simulink model "stage1_ball_joint_pd_uniform"  (R2025b)
settings: Solver=FixedStepDiscrete  StartTime=0.0  StopTime=stop_time_s  FixedStep=dt_sim  RelTol=1e-3
PostLoadFcn:
  | evalin('base', 'run(fullfile(fileparts(get_param(''stage1_ball_joint_pd_uniform'', ''FileName'')), ''init_stage1_ball_joint_pd_workspace.m''))')
InitFcn:
  | evalin('base', 'run(fullfile(fileparts(get_param(''stage1_ball_joint_pd_uniform'', ''FileName'')), ''init_stage1_ball_joint_pd_workspace.m''))')
values from neighbouring files (symbols this model uses):
  alpha_v = 1 - exp(-dt_ctrl / tau_v)    [init_stage1_ball_joint_pd_workspace.m]    (also in simulate_uniform_ball_joint_pd.m = 1 - exp(-dt_ctrl / params.tau_v))
  B_axis = 0.5    [init_stage1_ball_joint_pd_workspace.m]
  dt_ctrl = 1 / 60    (= 0.0166666666667)    [init_stage1_ball_joint_pd_workspace.m]    (also in simulate_uniform_ball_joint_pd.m = params.dt_ctrl)
  dt_sim = 1 / 120    (= 0.00833333333333)    [init_stage1_ball_joint_pd_workspace.m]    (also in simulate_uniform_ball_joint_pd.m = params.dt_sim)
  J_axis = 0.10    (= 0.1)    [init_stage1_ball_joint_pd_workspace.m]
  Kd = 10    [init_stage1_ball_joint_pd_workspace.m]    (also in plot_model725_trace_desired_vs_actual.m = 30)
  Kp = 120    [init_stage1_ball_joint_pd_workspace.m]    (also in plot_model725_trace_desired_vs_actual.m = 170)
  q_lower = [-0.7, -1.6, -0.5, -0.7, -1.6, -0.5]    [init_stage1_ball_joint_pd_workspace.m]    (also in plot_model725_trace_desired_vs_actual.m; simulate_uniform_ball_joint_pd.m = row_vector(params.q_lower))
  q_upper = [0.7, 0.5, 0.5, 0.7, 0.5, 0.5]    [init_stage1_ball_joint_pd_workspace.m]    (also in plot_model725_trace_desired_vs_actual.m; simulate_uniform_ball_joint_pd.m = row_vector(params.q_upper))
  qdot_max = 2    [init_stage1_ball_joint_pd_workspace.m]
  tau_load = 0    [init_stage1_ball_joint_pd_workspace.m]
  tau_max = 60    [init_stage1_ball_joint_pd_workspace.m]    (also in plot_model725_trace_desired_vs_actual.m)
undefined symbols (not defined in the file or in its folder): DiscIntNeverNeededParam
libraries: simulink x1
settings Model: Creator=ubuntu  LastModifiedBy=ubuntu

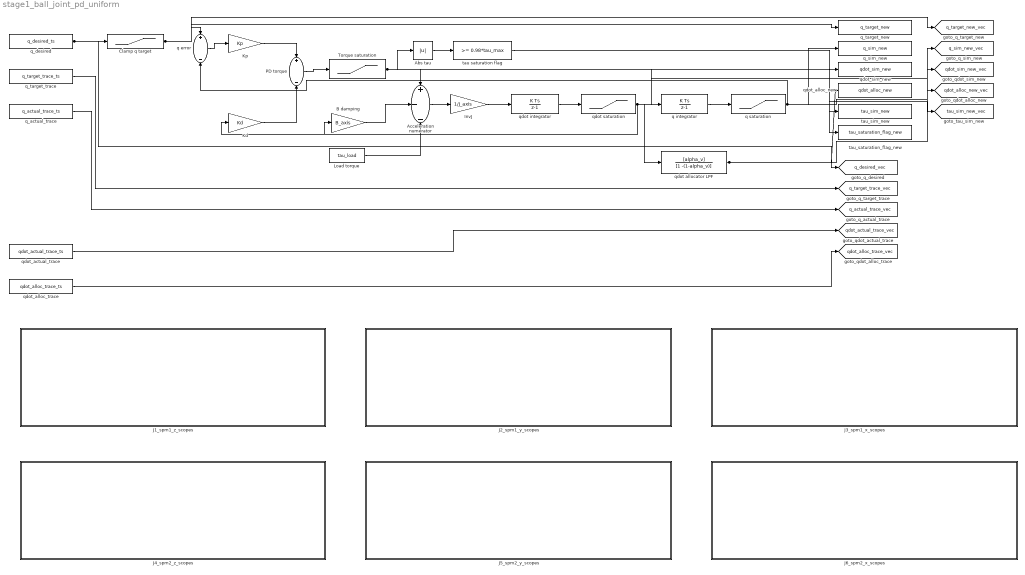
== system stage1_ball_joint_pd_uniform ==
  Abs tau : Abs  SaturateOnIntegerOverflow=off
  Acceleration numerator : Sum  Inputs=+--
  B damping : Gain  Gain=B_axis
  Clamp q target : Saturate  UpperLimit=q_upper  LowerLimit=q_lower
  InvJ : Gain  Gain=1/J_axis
  J1_spm1_z_scopes : Subsystem
  J2_spm1_y_scopes : Subsystem
  J3_spm1_x_scopes : Subsystem
  J4_spm2_z_scopes : Subsystem
  J5_spm2_y_scopes : Subsystem
  J6_spm2_x_scopes : Subsystem
  Kd : Gain  Gain=Kd
  Kp : Gain  Gain=Kp
  Load torque : Constant  Value=tau_load
  PD torque : Sum  Inputs=+-
  Torque saturation : Saturate  UpperLimit=tau_max  LowerLimit=-tau_max
  q error : Sum  Inputs=+-
  q integrator : DiscreteIntegrator  InitialCondition=zeros(1, 6)  SampleTime=dt_sim  ICPrevOutput=DiscIntNeverNeededParam  ICPrevScaledInput=DiscIntNeverNeededParam
  q saturation : Saturate  UpperLimit=q_upper  LowerLimit=q_lower
  q_actual_trace : FromWorkspace  VariableName=q_actual_trace_ts  SampleTime=dt_ctrl
  q_desired : FromWorkspace  VariableName=q_desired_ts  SampleTime=dt_ctrl
  q_sim_new : ToWorkspace  VariableName=q_sim_new  SaveFormat=Timeseries  SampleTime=-1
  q_target_new : ToWorkspace  VariableName=q_target_new  SaveFormat=Timeseries  SampleTime=-1
  q_target_trace : FromWorkspace  VariableName=q_target_trace_ts  SampleTime=dt_ctrl
  qdot allocator LPF : DiscreteTransferFcn  Numerator=[alpha_v]  Denominator=[1 -(1-alpha_v)]  SampleTime=dt_ctrl
  qdot integrator : DiscreteIntegrator  InitialCondition=zeros(1, 6)  SampleTime=dt_sim  ICPrevOutput=DiscIntNeverNeededParam  ICPrevScaledInput=DiscIntNeverNeededParam
  qdot saturation : Saturate  UpperLimit=qdot_max  LowerLimit=-qdot_max
  qdot_actual_trace : FromWorkspace  VariableName=qdot_actual_trace_ts  SampleTime=dt_ctrl
  qdot_alloc_new : ToWorkspace  VariableName=qdot_alloc_new  SaveFormat=Timeseries  SampleTime=-1
  qdot_alloc_trace : FromWorkspace  VariableName=qdot_alloc_trace_ts  SampleTime=dt_ctrl
  qdot_sim_new : ToWorkspace  VariableName=qdot_sim_new  SaveFormat=Timeseries  SampleTime=-1
  tau saturation flag : simulink/Logic and Bit Operations/Compare To Constant  relop=>=  const=0.98*tau_max  OutDataTypeStr=boolean
  tau_saturation_flag_new : ToWorkspace  VariableName=tau_saturation_flag_new  SaveFormat=Timeseries  SampleTime=-1
  tau_sim_new : ToWorkspace  VariableName=tau_sim_new  SaveFormat=Timeseries  SampleTime=-1
  tag scope: q_actual_trace_vec=global, q_desired_vec=global, q_sim_new_vec=global, q_target_new_vec=global, q_target_trace_vec=global, qdot_actual_trace_vec=global, qdot_alloc_new_vec=global, qdot_alloc_trace_vec=global, qdot_sim_new_vec=global, tau_sim_new_vec=global
  wires:
  q_desired/1 -> Clamp q target/1, [q_desired_vec]
  Clamp q target/1 -> q error/1, q_target_new/1, [q_target_new_vec]
  q saturation/1 -> q error/2, q_sim_new/1, [q_sim_new_vec]
  q error/1 -> Kp/1
  Kp/1 -> PD torque/1
  qdot saturation/1 -> Kd/1, B damping/1, q integrator/1, qdot allocator LPF/1, qdot_sim_new/1, [qdot_sim_new_vec]
  Kd/1 -> PD torque/2
  PD torque/1 -> Torque saturation/1
  Torque saturation/1 -> Acceleration numerator/1, Abs tau/1, tau_sim_new/1, [tau_sim_new_vec]
  B damping/1 -> Acceleration numerator/2
  Load torque/1 -> Acceleration numerator/3
  Acceleration numerator/1 -> InvJ/1
  InvJ/1 -> qdot integrator/1
  qdot integrator/1 -> qdot saturation/1
  q integrator/1 -> q saturation/1
  Abs tau/1 -> tau saturation flag/1
  qdot allocator LPF/1 -> qdot_alloc_new/1, [qdot_alloc_new_vec]
  tau saturation flag/1 -> tau_saturation_flag_new/1
  q_target_trace/1 -> [q_target_trace_vec]
  q_actual_trace/1 -> [q_actual_trace_vec]
  qdot_actual_trace/1 -> [qdot_actual_trace_vec]
  qdot_alloc_trace/1 -> [qdot_alloc_trace_vec]

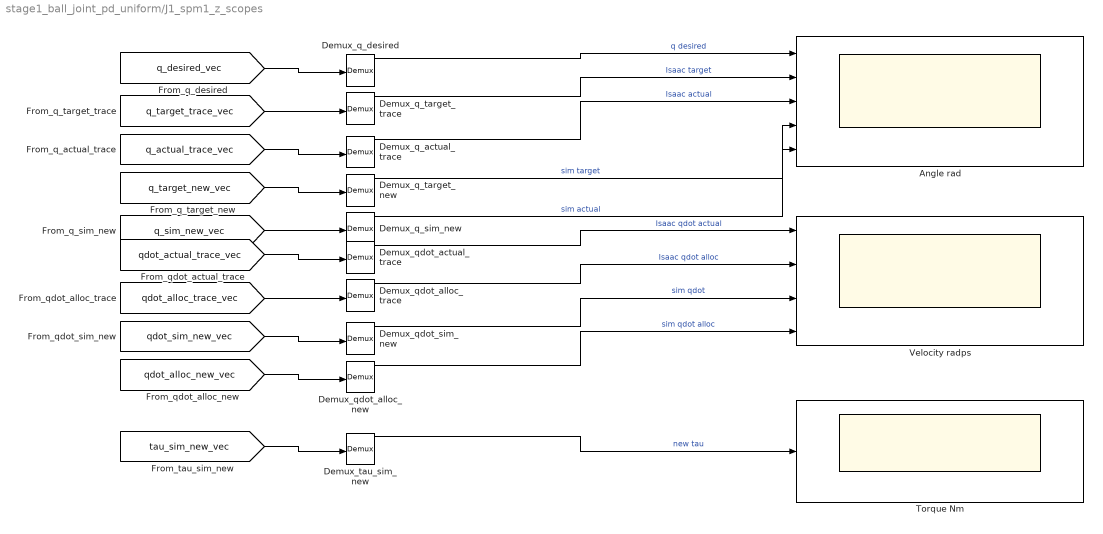
== system stage1_ball_joint_pd_uniform/J1_spm1_z_scopes ==
  Angle rad : Scope  NumInputPorts=5
      settings: MaximizeAxes=On  Title=Angle response  YLabel=Angle (rad)
  Demux_q_actual_trace : Demux  Outputs=6
  Demux_q_desired : Demux  Outputs=6
  Demux_q_sim_new : Demux  Outputs=6
  Demux_q_target_new : Demux  Outputs=6
  Demux_q_target_trace : Demux  Outputs=6
  Demux_qdot_actual_trace : Demux  Outputs=6
  Demux_qdot_alloc_new : Demux  Outputs=6
  Demux_qdot_alloc_trace : Demux  Outputs=6
  Demux_qdot_sim_new : Demux  Outputs=6
  Demux_tau_sim_new : Demux  Outputs=6
  Torque Nm : Scope
      settings: MaximizeAxes=On  Title=Torque command  YLabel=Torque (N*m)
  Velocity radps : Scope  NumInputPorts=4
      settings: MaximizeAxes=On  Title=Velocity response  YLabel=Velocity (rad/s)
  wires:
  [q_desired_vec] -> Demux_q_desired/1
  Demux_q_desired/1 -> Angle rad/1  "q desired"
  [q_target_trace_vec] -> Demux_q_target_trace/1
  Demux_q_target_trace/1 -> Angle rad/2  "Isaac target"
  [q_actual_trace_vec] -> Demux_q_actual_trace/1
  Demux_q_actual_trace/1 -> Angle rad/3  "Isaac actual"
  [q_target_new_vec] -> Demux_q_target_new/1
  Demux_q_target_new/1 -> Angle rad/4  "sim target"
  [q_sim_new_vec] -> Demux_q_sim_new/1
  Demux_q_sim_new/1 -> Angle rad/5  "sim actual"
  [qdot_actual_trace_vec] -> Demux_qdot_actual_trace/1
  Demux_qdot_actual_trace/1 -> Velocity radps/1  "Isaac qdot actual"
  [qdot_alloc_trace_vec] -> Demux_qdot_alloc_trace/1
  Demux_qdot_alloc_trace/1 -> Velocity radps/2  "Isaac qdot alloc"
  [qdot_sim_new_vec] -> Demux_qdot_sim_new/1
  Demux_qdot_sim_new/1 -> Velocity radps/3  "sim qdot"
  [qdot_alloc_new_vec] -> Demux_qdot_alloc_new/1
  Demux_qdot_alloc_new/1 -> Velocity radps/4  "sim qdot alloc"
  [tau_sim_new_vec] -> Demux_tau_sim_new/1
  Demux_tau_sim_new/1 -> Torque Nm/1  "new tau"

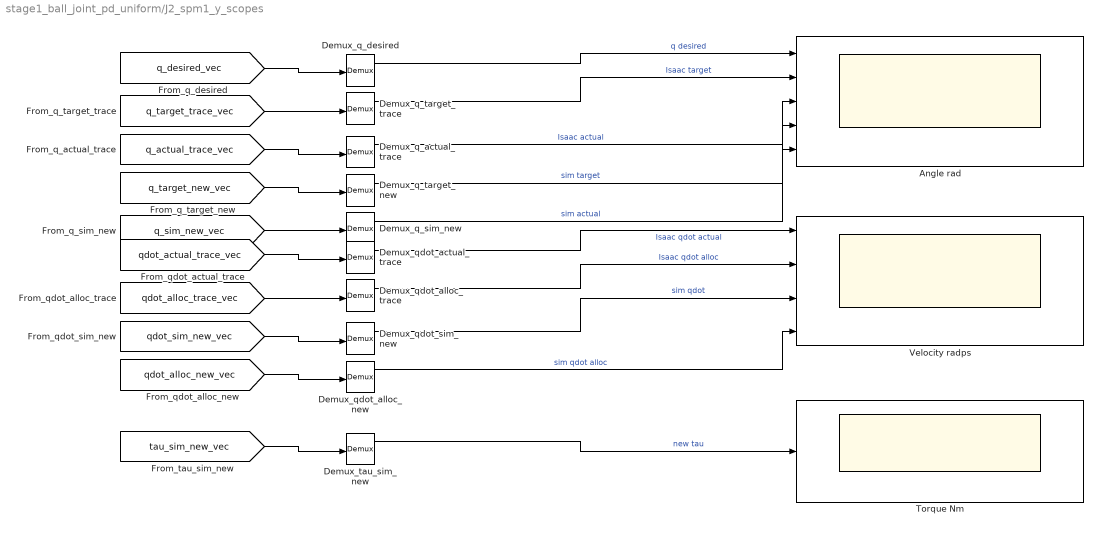
== system stage1_ball_joint_pd_uniform/J2_spm1_y_scopes ==
  Angle rad : Scope  NumInputPorts=5
      settings: MaximizeAxes=On  Title=Angle response  YLabel=Angle (rad)
  Demux_q_actual_trace : Demux  Outputs=6
  Demux_q_desired : Demux  Outputs=6
  Demux_q_sim_new : Demux  Outputs=6
  Demux_q_target_new : Demux  Outputs=6
  Demux_q_target_trace : Demux  Outputs=6
  Demux_qdot_actual_trace : Demux  Outputs=6
  Demux_qdot_alloc_new : Demux  Outputs=6
  Demux_qdot_alloc_trace : Demux  Outputs=6
  Demux_qdot_sim_new : Demux  Outputs=6
  Demux_tau_sim_new : Demux  Outputs=6
  Torque Nm : Scope
      settings: MaximizeAxes=On  Title=Torque command  YLabel=Torque (N*m)
  Velocity radps : Scope  NumInputPorts=4
      settings: MaximizeAxes=On  Title=Velocity response  YLabel=Velocity (rad/s)
  wires:
  [q_desired_vec] -> Demux_q_desired/1
  Demux_q_desired/2 -> Angle rad/1  "q desired"
  [q_target_trace_vec] -> Demux_q_target_trace/1
  Demux_q_target_trace/2 -> Angle rad/2  "Isaac target"
  [q_actual_trace_vec] -> Demux_q_actual_trace/1
  Demux_q_actual_trace/2 -> Angle rad/3  "Isaac actual"
  [q_target_new_vec] -> Demux_q_target_new/1
  Demux_q_target_new/2 -> Angle rad/4  "sim target"
  [q_sim_new_vec] -> Demux_q_sim_new/1
  Demux_q_sim_new/2 -> Angle rad/5  "sim actual"
  [qdot_actual_trace_vec] -> Demux_qdot_actual_trace/1
  Demux_qdot_actual_trace/2 -> Velocity radps/1  "Isaac qdot actual"
  [qdot_alloc_trace_vec] -> Demux_qdot_alloc_trace/1
  Demux_qdot_alloc_trace/2 -> Velocity radps/2  "Isaac qdot alloc"
  [qdot_sim_new_vec] -> Demux_qdot_sim_new/1
  Demux_qdot_sim_new/2 -> Velocity radps/3  "sim qdot"
  [qdot_alloc_new_vec] -> Demux_qdot_alloc_new/1
  Demux_qdot_alloc_new/2 -> Velocity radps/4  "sim qdot alloc"
  [tau_sim_new_vec] -> Demux_tau_sim_new/1
  Demux_tau_sim_new/2 -> Torque Nm/1  "new tau"

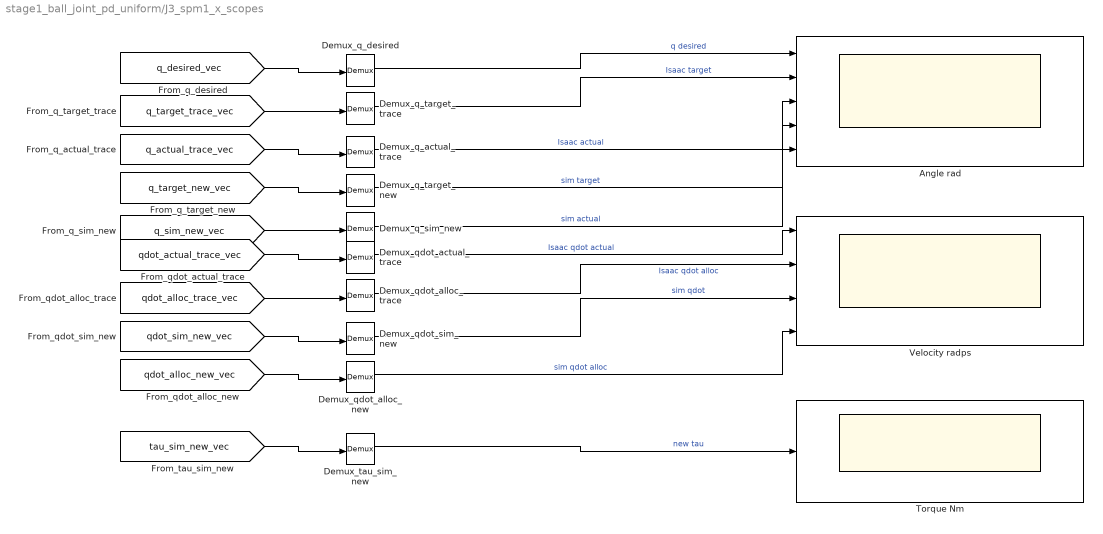
== system stage1_ball_joint_pd_uniform/J3_spm1_x_scopes ==
  Angle rad : Scope  NumInputPorts=5
      settings: MaximizeAxes=On  Title=Angle response  YLabel=Angle (rad)
  Demux_q_actual_trace : Demux  Outputs=6
  Demux_q_desired : Demux  Outputs=6
  Demux_q_sim_new : Demux  Outputs=6
  Demux_q_target_new : Demux  Outputs=6
  Demux_q_target_trace : Demux  Outputs=6
  Demux_qdot_actual_trace : Demux  Outputs=6
  Demux_qdot_alloc_new : Demux  Outputs=6
  Demux_qdot_alloc_trace : Demux  Outputs=6
  Demux_qdot_sim_new : Demux  Outputs=6
  Demux_tau_sim_new : Demux  Outputs=6
  Torque Nm : Scope
      settings: MaximizeAxes=On  Title=Torque command  YLabel=Torque (N*m)
  Velocity radps : Scope  NumInputPorts=4
      settings: MaximizeAxes=On  Title=Velocity response  YLabel=Velocity (rad/s)
  wires:
  [q_desired_vec] -> Demux_q_desired/1
  Demux_q_desired/3 -> Angle rad/1  "q desired"
  [q_target_trace_vec] -> Demux_q_target_trace/1
  Demux_q_target_trace/3 -> Angle rad/2  "Isaac target"
  [q_actual_trace_vec] -> Demux_q_actual_trace/1
  Demux_q_actual_trace/3 -> Angle rad/3  "Isaac actual"
  [q_target_new_vec] -> Demux_q_target_new/1
  Demux_q_target_new/3 -> Angle rad/4  "sim target"
  [q_sim_new_vec] -> Demux_q_sim_new/1
  Demux_q_sim_new/3 -> Angle rad/5  "sim actual"
  [qdot_actual_trace_vec] -> Demux_qdot_actual_trace/1
  Demux_qdot_actual_trace/3 -> Velocity radps/1  "Isaac qdot actual"
  [qdot_alloc_trace_vec] -> Demux_qdot_alloc_trace/1
  Demux_qdot_alloc_trace/3 -> Velocity radps/2  "Isaac qdot alloc"
  [qdot_sim_new_vec] -> Demux_qdot_sim_new/1
  Demux_qdot_sim_new/3 -> Velocity radps/3  "sim qdot"
  [qdot_alloc_new_vec] -> Demux_qdot_alloc_new/1
  Demux_qdot_alloc_new/3 -> Velocity radps/4  "sim qdot alloc"
  [tau_sim_new_vec] -> Demux_tau_sim_new/1
  Demux_tau_sim_new/3 -> Torque Nm/1  "new tau"

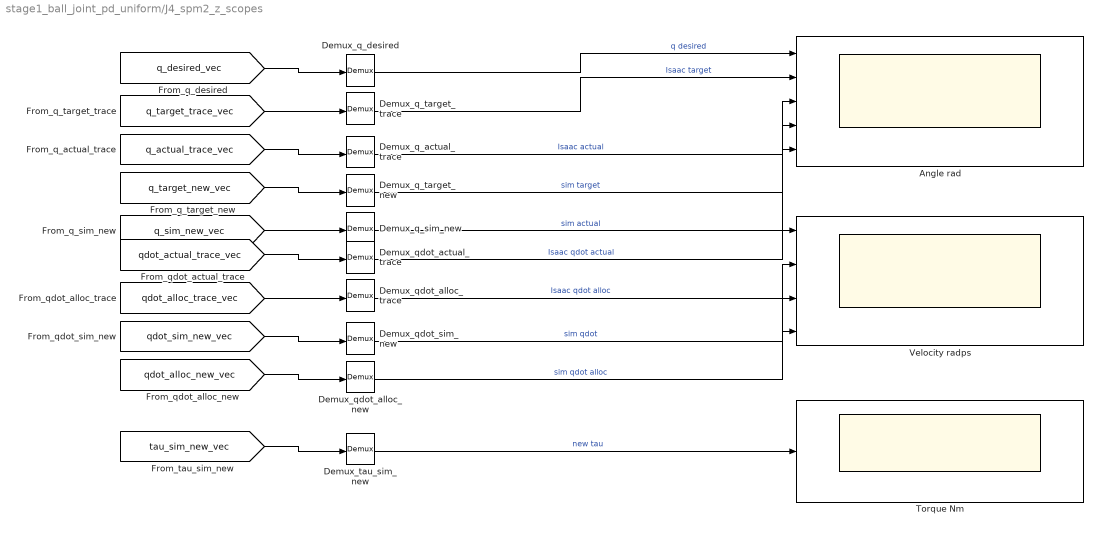
== system stage1_ball_joint_pd_uniform/J4_spm2_z_scopes ==
  Angle rad : Scope  NumInputPorts=5
      settings: MaximizeAxes=On  Title=Angle response  YLabel=Angle (rad)
  Demux_q_actual_trace : Demux  Outputs=6
  Demux_q_desired : Demux  Outputs=6
  Demux_q_sim_new : Demux  Outputs=6
  Demux_q_target_new : Demux  Outputs=6
  Demux_q_target_trace : Demux  Outputs=6
  Demux_qdot_actual_trace : Demux  Outputs=6
  Demux_qdot_alloc_new : Demux  Outputs=6
  Demux_qdot_alloc_trace : Demux  Outputs=6
  Demux_qdot_sim_new : Demux  Outputs=6
  Demux_tau_sim_new : Demux  Outputs=6
  Torque Nm : Scope
      settings: MaximizeAxes=On  Title=Torque command  YLabel=Torque (N*m)
  Velocity radps : Scope  NumInputPorts=4
      settings: MaximizeAxes=On  Title=Velocity response  YLabel=Velocity (rad/s)
  wires:
  [q_desired_vec] -> Demux_q_desired/1
  Demux_q_desired/4 -> Angle rad/1  "q desired"
  [q_target_trace_vec] -> Demux_q_target_trace/1
  Demux_q_target_trace/4 -> Angle rad/2  "Isaac target"
  [q_actual_trace_vec] -> Demux_q_actual_trace/1
  Demux_q_actual_trace/4 -> Angle rad/3  "Isaac actual"
  [q_target_new_vec] -> Demux_q_target_new/1
  Demux_q_target_new/4 -> Angle rad/4  "sim target"
  [q_sim_new_vec] -> Demux_q_sim_new/1
  Demux_q_sim_new/4 -> Angle rad/5  "sim actual"
  [qdot_actual_trace_vec] -> Demux_qdot_actual_trace/1
  Demux_qdot_actual_trace/4 -> Velocity radps/1  "Isaac qdot actual"
  [qdot_alloc_trace_vec] -> Demux_qdot_alloc_trace/1
  Demux_qdot_alloc_trace/4 -> Velocity radps/2  "Isaac qdot alloc"
  [qdot_sim_new_vec] -> Demux_qdot_sim_new/1
  Demux_qdot_sim_new/4 -> Velocity radps/3  "sim qdot"
  [qdot_alloc_new_vec] -> Demux_qdot_alloc_new/1
  Demux_qdot_alloc_new/4 -> Velocity radps/4  "sim qdot alloc"
  [tau_sim_new_vec] -> Demux_tau_sim_new/1
  Demux_tau_sim_new/4 -> Torque Nm/1  "new tau"

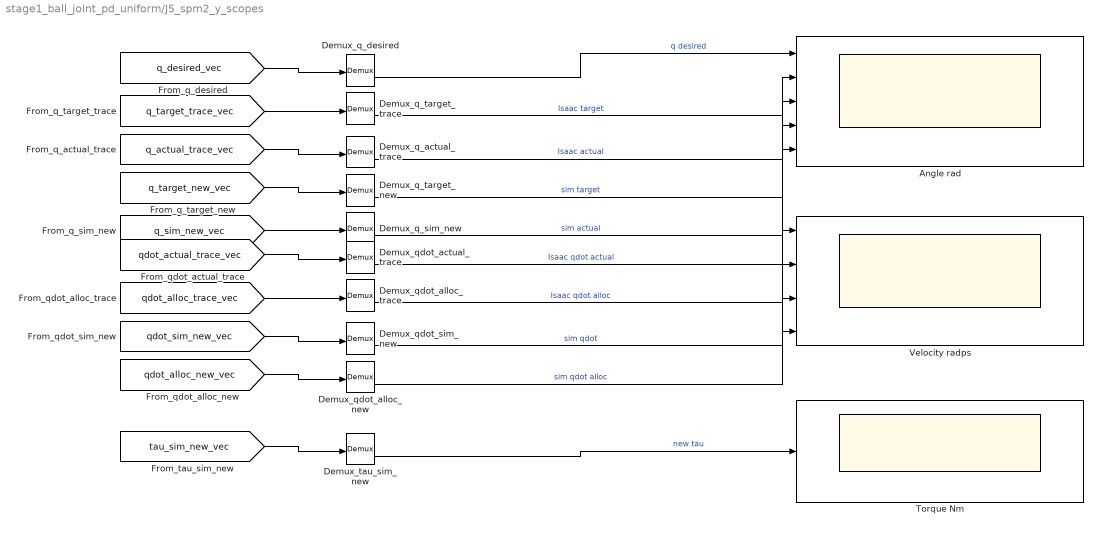
== system stage1_ball_joint_pd_uniform/J5_spm2_y_scopes ==
  Angle rad : Scope  NumInputPorts=5
      settings: MaximizeAxes=On  Title=Angle response  YLabel=Angle (rad)
  Demux_q_actual_trace : Demux  Outputs=6
  Demux_q_desired : Demux  Outputs=6
  Demux_q_sim_new : Demux  Outputs=6
  Demux_q_target_new : Demux  Outputs=6
  Demux_q_target_trace : Demux  Outputs=6
  Demux_qdot_actual_trace : Demux  Outputs=6
  Demux_qdot_alloc_new : Demux  Outputs=6
  Demux_qdot_alloc_trace : Demux  Outputs=6
  Demux_qdot_sim_new : Demux  Outputs=6
  Demux_tau_sim_new : Demux  Outputs=6
  Torque Nm : Scope
      settings: MaximizeAxes=On  Title=Torque command  YLabel=Torque (N*m)
  Velocity radps : Scope  NumInputPorts=4
      settings: MaximizeAxes=On  Title=Velocity response  YLabel=Velocity (rad/s)
  wires:
  [q_desired_vec] -> Demux_q_desired/1
  Demux_q_desired/5 -> Angle rad/1  "q desired"
  [q_target_trace_vec] -> Demux_q_target_trace/1
  Demux_q_target_trace/5 -> Angle rad/2  "Isaac target"
  [q_actual_trace_vec] -> Demux_q_actual_trace/1
  Demux_q_actual_trace/5 -> Angle rad/3  "Isaac actual"
  [q_target_new_vec] -> Demux_q_target_new/1
  Demux_q_target_new/5 -> Angle rad/4  "sim target"
  [q_sim_new_vec] -> Demux_q_sim_new/1
  Demux_q_sim_new/5 -> Angle rad/5  "sim actual"
  [qdot_actual_trace_vec] -> Demux_qdot_actual_trace/1
  Demux_qdot_actual_trace/5 -> Velocity radps/1  "Isaac qdot actual"
  [qdot_alloc_trace_vec] -> Demux_qdot_alloc_trace/1
  Demux_qdot_alloc_trace/5 -> Velocity radps/2  "Isaac qdot alloc"
  [qdot_sim_new_vec] -> Demux_qdot_sim_new/1
  Demux_qdot_sim_new/5 -> Velocity radps/3  "sim qdot"
  [qdot_alloc_new_vec] -> Demux_qdot_alloc_new/1
  Demux_qdot_alloc_new/5 -> Velocity radps/4  "sim qdot alloc"
  [tau_sim_new_vec] -> Demux_tau_sim_new/1
  Demux_tau_sim_new/5 -> Torque Nm/1  "new tau"

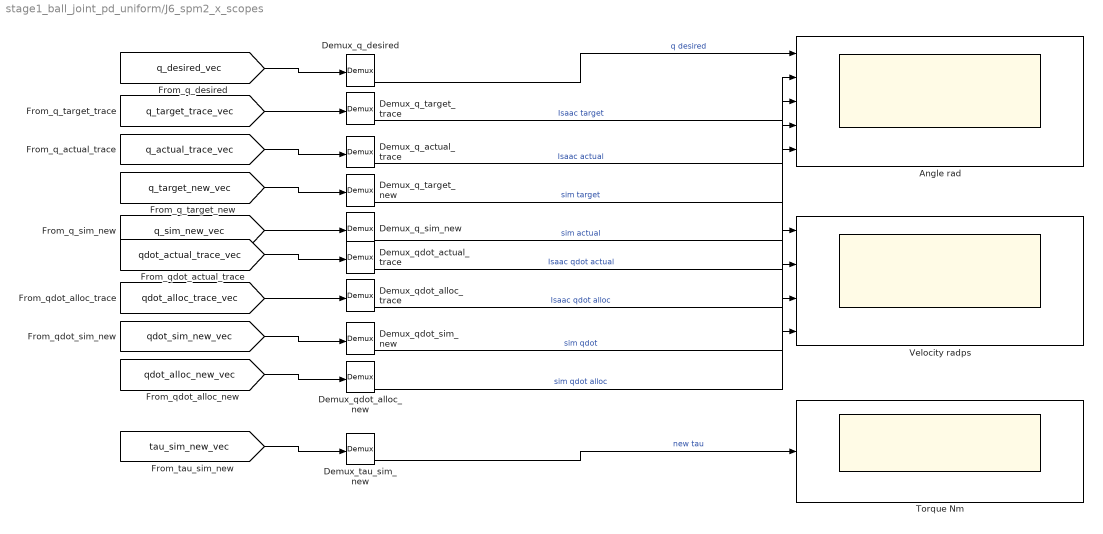
== system stage1_ball_joint_pd_uniform/J6_spm2_x_scopes ==
  Angle rad : Scope  NumInputPorts=5
      settings: MaximizeAxes=On  Title=Angle response  YLabel=Angle (rad)
  Demux_q_actual_trace : Demux  Outputs=6
  Demux_q_desired : Demux  Outputs=6
  Demux_q_sim_new : Demux  Outputs=6
  Demux_q_target_new : Demux  Outputs=6
  Demux_q_target_trace : Demux  Outputs=6
  Demux_qdot_actual_trace : Demux  Outputs=6
  Demux_qdot_alloc_new : Demux  Outputs=6
  Demux_qdot_alloc_trace : Demux  Outputs=6
  Demux_qdot_sim_new : Demux  Outputs=6
  Demux_tau_sim_new : Demux  Outputs=6
  Torque Nm : Scope
      settings: MaximizeAxes=On  Title=Torque command  YLabel=Torque (N*m)
  Velocity radps : Scope  NumInputPorts=4
      settings: MaximizeAxes=On  Title=Velocity response  YLabel=Velocity (rad/s)
  wires:
  [q_desired_vec] -> Demux_q_desired/1
  Demux_q_desired/6 -> Angle rad/1  "q desired"
  [q_target_trace_vec] -> Demux_q_target_trace/1
  Demux_q_target_trace/6 -> Angle rad/2  "Isaac target"
  [q_actual_trace_vec] -> Demux_q_actual_trace/1
  Demux_q_actual_trace/6 -> Angle rad/3  "Isaac actual"
  [q_target_new_vec] -> Demux_q_target_new/1
  Demux_q_target_new/6 -> Angle rad/4  "sim target"
  [q_sim_new_vec] -> Demux_q_sim_new/1
  Demux_q_sim_new/6 -> Angle rad/5  "sim actual"
  [qdot_actual_trace_vec] -> Demux_qdot_actual_trace/1
  Demux_qdot_actual_trace/6 -> Velocity radps/1  "Isaac qdot actual"
  [qdot_alloc_trace_vec] -> Demux_qdot_alloc_trace/1
  Demux_qdot_alloc_trace/6 -> Velocity radps/2  "Isaac qdot alloc"
  [qdot_sim_new_vec] -> Demux_qdot_sim_new/1
  Demux_qdot_sim_new/6 -> Velocity radps/3  "sim qdot"
  [qdot_alloc_new_vec] -> Demux_qdot_alloc_new/1
  Demux_qdot_alloc_new/6 -> Velocity radps/4  "sim qdot alloc"
  [tau_sim_new_vec] -> Demux_tau_sim_new/1
  Demux_tau_sim_new/6 -> Torque Nm/1  "new tau"
